simulink model "demo_cls1"  (R2016b)
settings: Solver=FixedStepDiscrete  StartTime=0.0  StopTime=10.0  FixedStep=0.01  RelTol=1e-3
settings Model: Creator=Borja Martos  LastModifiedBy=Borja Martos

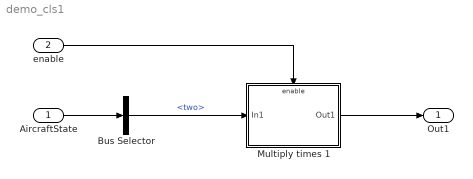
== system demo_cls1 ==
  AircraftState : Inport  OutDataTypeStr=Bus: INPUTS
  enable : Inport  Port=2  OutDataTypeStr=boolean
  Bus Selector : BusSelector  OutputSignals=two
  Multiply times 1 : Subsystem
  Out1 : Outport
  wires:
  enable/1 -> Multiply times 1/Enable
  AircraftState/1 -> Bus Selector/1
  Bus Selector/1 -> Multiply times 1/1(In1)  "<two>"
  Multiply times 1/1(Out1) -> Out1/1

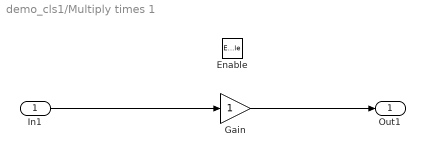
== system demo_cls1/Multiply times 1 ==
  In1 : Inport
  Enable : EnablePort  StatesWhenEnabling=reset
  Gain : Gain
  Out1 : Outport
  wires:
  Gain/1 -> Out1/1
  In1/1 -> Gain/1
